simulink model "Demo_PreScanCarSim3D_ExtFMU_cs"  (Simulink 8.6)
settings: Solver=ode5  SolverMode=SingleTasking  StartTime=0.0  StopTime=68  FixedStep=1/1000  RelTol=1e-3
PreLoadFcn:
  | mbxruntime.callbacks.PreLoadFcn(bdroot);
  | check_NUTS_defined;
  | 
  | assignin('base',['model_closed_' bdroot],false);
PostLoadFcn:
  | mbxruntime.callbacks.PostLoadFcn(bdroot);
InitFcn:
  | mbxruntime.callbacks.InitFcn(bdroot);
StartFcn:
  | mbxruntime.callbacks.StartFcn(bdroot);
StopFcn:
  | mbxruntime.callbacks.StopFcn(bdroot);
undefined symbols (not defined in the file): DiscIntNeverNeededParam, mbxruntime, tabledata, warningInitialVelocity, x0, x_ini_VRML, y_ini_VRML, z_ini_VRML
libraries: PreScanSimulinkLibrary x15, simulink_extras x8, simulink x5, PreScanCarSimLibrary x1
(part 2 of 11)

== system Demo_PreScanCarSim3D_ExtFMU_cs/TrafficLightRoadSideNL_1 ==
  DISABLED : Subsystem  VariantControl=off
  ENABLED : Subsystem  VariantControl=on
  VISUCasingLights_TrafficLightRoadSideNL_1 : Outport  Tag=outport/VisuCasingLights  SampleTime=50/1000

== system Demo_PreScanCarSim3D_ExtFMU_cs/TrafficLightRoadSideNL_2 ==
  DISABLED : Subsystem  VariantControl=off
  ENABLED : Subsystem  VariantControl=on
  VISUCasingLights_TrafficLightRoadSideNL_2 : Outport  Tag=outport/VisuCasingLights  SampleTime=50/1000

== system Demo_PreScanCarSim3D_ExtFMU_cs/TrafficLightRoadSideNL_3 ==
  DISABLED : Subsystem  VariantControl=off
  ENABLED : Subsystem  VariantControl=on
  VISUCasingLights_TrafficLightRoadSideNL_3 : Outport  Tag=outport/VisuCasingLights  SampleTime=50/1000

== system Demo_PreScanCarSim3D_ExtFMU_cs/TrafficLightRoadSideNL_5 ==
  DISABLED : Subsystem  VariantControl=off
  ENABLED : Subsystem  VariantControl=on
  VISUCasingLights_TrafficLightRoadSideNL_5 : Outport  Tag=outport/VisuCasingLights  SampleTime=50/1000

== system Demo_PreScanCarSim3D_ExtFMU_cs/TrafficLightRoadSideNL_6 ==
  DISABLED : Subsystem  VariantControl=off
  ENABLED : Subsystem  VariantControl=on
  VISUCasingLights_TrafficLightRoadSideNL_6 : Outport  Tag=outport/VisuCasingLights  SampleTime=50/1000

== system Demo_PreScanCarSim3D_ExtFMU_cs/TrafficLightRoadSideNL_7 ==
  DISABLED : Subsystem  VariantControl=off
  ENABLED : Subsystem  VariantControl=on
  VISUCasingLights_TrafficLightRoadSideNL_7 : Outport  Tag=outport/VisuCasingLights  SampleTime=50/1000

== system Demo_PreScanCarSim3D_ExtFMU_cs/VISUCasingLights_TrafficLightRoadSideNL_1 ==
  VISUCasingLights_TrafficLightRoadSideNL_1 : Inport  Tag=inport/VisuCasingLights  SampleTime=50/1000  BusOutputAsStruct=on
  DISABLED : Subsystem  VariantControl=off
  ENABLED : Subsystem  VariantControl=on

== system Demo_PreScanCarSim3D_ExtFMU_cs/VISUCasingLights_TrafficLightRoadSideNL_2 ==
  VISUCasingLights_TrafficLightRoadSideNL_2 : Inport  Tag=inport/VisuCasingLights  SampleTime=50/1000  BusOutputAsStruct=on
  DISABLED : Subsystem  VariantControl=off
  ENABLED : Subsystem  VariantControl=on

== system Demo_PreScanCarSim3D_ExtFMU_cs/VISUCasingLights_TrafficLightRoadSideNL_3 ==
  VISUCasingLights_TrafficLightRoadSideNL_3 : Inport  Tag=inport/VisuCasingLights  SampleTime=50/1000  BusOutputAsStruct=on
  DISABLED : Subsystem  VariantControl=off
  ENABLED : Subsystem  VariantControl=on

== system Demo_PreScanCarSim3D_ExtFMU_cs/VISUCasingLights_TrafficLightRoadSideNL_5 ==
  VISUCasingLights_TrafficLightRoadSideNL_5 : Inport  Tag=inport/VisuCasingLights  SampleTime=50/1000  BusOutputAsStruct=on
  DISABLED : Subsystem  VariantControl=off
  ENABLED : Subsystem  VariantControl=on

== system Demo_PreScanCarSim3D_ExtFMU_cs/VISUCasingLights_TrafficLightRoadSideNL_6 ==
  VISUCasingLights_TrafficLightRoadSideNL_6 : Inport  Tag=inport/VisuCasingLights  SampleTime=50/1000  BusOutputAsStruct=on
  DISABLED : Subsystem  VariantControl=off
  ENABLED : Subsystem  VariantControl=on

== system Demo_PreScanCarSim3D_ExtFMU_cs/VISUCasingLights_TrafficLightRoadSideNL_7 ==
  VISUCasingLights_TrafficLightRoadSideNL_7 : Inport  Tag=inport/VisuCasingLights  SampleTime=50/1000  BusOutputAsStruct=on
  DISABLED : Subsystem  VariantControl=off
  ENABLED : Subsystem  VariantControl=on

== system Demo_PreScanCarSim3D_ExtFMU_cs/VISUMatrixSignLights_HighwayOverhang_1 ==
  VISUMatrixSignLights_HighwayOverhang_1 : Inport  Tag=inport/VisuMatrixSignLights  SampleTime=50/1000  BusOutputAsStruct=on
  DISABLED : Subsystem  VariantControl=off
  ENABLED : Subsystem  VariantControl=on

== system Demo_PreScanCarSim3D_ExtFMU_cs/VISUMatrixSignLights_HighwayOverhang_2 ==
  VISUMatrixSignLights_HighwayOverhang_2 : Inport  Tag=inport/VisuMatrixSignLights  SampleTime=50/1000  BusOutputAsStruct=on
  DISABLED : Subsystem  VariantControl=off
  ENABLED : Subsystem  VariantControl=on

== system Demo_PreScanCarSim3D_ExtFMU_cs/VISUMatrixSignLights_HighwayOverhang_3 ==
  VISUMatrixSignLights_HighwayOverhang_3 : Inport  Tag=inport/VisuMatrixSignLights  SampleTime=50/1000  BusOutputAsStruct=on
  DISABLED : Subsystem  VariantControl=off
  ENABLED : Subsystem  VariantControl=on

== system Demo_PreScanCarSim3D_ExtFMU_cs/VISUMatrixSignLights_HighwayOverhang_5 ==
  VISUMatrixSignLights_HighwayOverhang_5 : Inport  Tag=inport/VisuMatrixSignLights  SampleTime=50/1000  BusOutputAsStruct=on
  DISABLED : Subsystem  VariantControl=off
  ENABLED : Subsystem  VariantControl=on

== system Demo_PreScanCarSim3D_ExtFMU_cs/VISUMatrixSign_HighwayOverhang_1 ==
  VISUMatrixSign_HighwayOverhang_1 : Inport  Tag=inport/VisuMatrixSign  SampleTime=50/1000  BusOutputAsStruct=on
  DISABLED : Subsystem  VariantControl=off
  ENABLED : Subsystem  VariantControl=on

== system Demo_PreScanCarSim3D_ExtFMU_cs/VISUMatrixSign_HighwayOverhang_2 ==
  VISUMatrixSign_HighwayOverhang_2 : Inport  Tag=inport/VisuMatrixSign  SampleTime=50/1000  BusOutputAsStruct=on
  DISABLED : Subsystem  VariantControl=off
  ENABLED : Subsystem  VariantControl=on

== system Demo_PreScanCarSim3D_ExtFMU_cs/VISUMatrixSign_HighwayOverhang_3 ==
  VISUMatrixSign_HighwayOverhang_3 : Inport  Tag=inport/VisuMatrixSign  SampleTime=50/1000  BusOutputAsStruct=on
  DISABLED : Subsystem  VariantControl=off
  ENABLED : Subsystem  VariantControl=on

== system Demo_PreScanCarSim3D_ExtFMU_cs/VISUMatrixSign_HighwayOverhang_5 ==
  VISUMatrixSign_HighwayOverhang_5 : Inport  Tag=inport/VisuMatrixSign  SampleTime=50/1000  BusOutputAsStruct=on
  DISABLED : Subsystem  VariantControl=off
  ENABLED : Subsystem  VariantControl=on

== system Demo_PreScanCarSim3D_ExtFMU_cs/VISUWheelsCarSim_Audi_A8_1 ==
  VISUWheelsCarSim_Audi_A8_1 : Inport  Tag=inport/VisuWheels  SampleTime=50/1000  BusOutputAsStruct=on
  DISABLED : Subsystem  VariantControl=off
  ENABLED : Subsystem  VariantControl=on

== system Demo_PreScanCarSim3D_ExtFMU_cs/Audi_A8_1/DISABLED ==
  SELF_Audi_A8_1 : Inport  Tag=inport/SelfPort  OutDataTypeStr=Bus: PRESCAN_SELFSENSORDATA  PortDimensions=1  SampleTime=50/1000  BusOutputAsStruct=on
  FromCarSimFMU : Inport  Tag=inport/  Port=2  BusOutputAsStruct=on
  GND1 : Subsystem
  GND2 : Ground
  GND3 : Ground
  TRM1 : Terminator
  TRM2 : Terminator
  STATE_Audi_A8_1_bus : Outport  Tag=outport/StatePort  OutDataTypeStr=Bus: PRESCAN_STATEACTUATORDATA  PortDimensions=1  SampleTime=50/1000
  VISUWheelsCarSim_Audi_A8_1 : Outport  Tag=outport/VisuWheels  Port=2  SampleTime=50/1000
  ToCarSimFMU : Outport  Tag=outport/  Port=3
  wires:
  SELF_Audi_A8_1/1 -> TRM1/1
  FromCarSimFMU/1 -> TRM2/1
  GND1/1(bus) -> STATE_Audi_A8_1_bus/1
  GND2/1 -> VISUWheelsCarSim_Audi_A8_1/1
  GND3/1 -> ToCarSimFMU/1

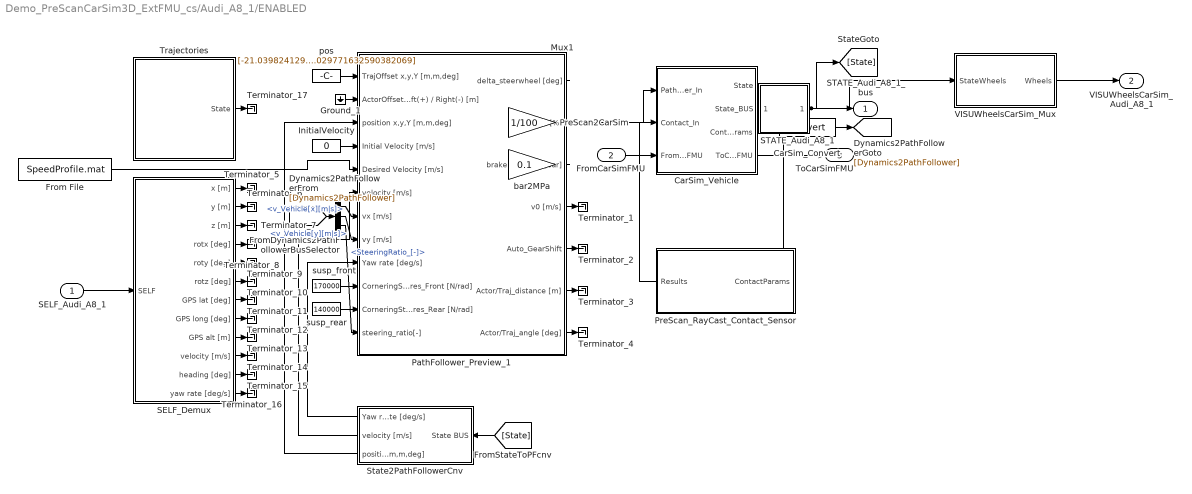
== system Demo_PreScanCarSim3D_ExtFMU_cs/Audi_A8_1/ENABLED ==
  SELF_Audi_A8_1 : Inport  Tag=inport/SelfPort  OutDataTypeStr=Bus: PRESCAN_SELFSENSORDATA  PortDimensions=1  SampleTime=50/1000  BusOutputAsStruct=on
  FromCarSimFMU : Inport  Port=2
  CarSim_Convert : PreScanCarSimLibrary/Convert  Tag=ConvertCarSim  SystemSampleTime=-1
  CarSim_Vehicle : Subsystem  Tag=UserSpecified_Subsys  Description=.\Connection2CarSimFMU.mdl  mask(User specified subsystem){update=off, sourcefilename=.\Connection2CarSimFMU.mdl}
      mask prompts: update "Update (default: not checked)"; sourcefilename "Source file name"
      mask help:
      | A User-specified model may be selected as Controller or Dynamics of the vehicle. PreScan will copy the contents of the User-specified model into the user-specified model block.
      |
      | If update checkbox is checked the current user-specified model block will be deleted and will be REPLACED by (new) user specified model blocks. So, the current user specified model elements will be lost.
      |
      | Warning: If a new user-specified model is selected in the GUI, the user-specified model will be replaced.
      settings: DeleteFcn=PreScanBlockDeleteFcn;
      mask Help: eval('openHelp(227)')
      mask Display: userSpecifiedDynamics_mask_display();
  From File : FromFile  FileName=SpeedProfile.mat  SampleTime=eval(get_param(bdroot,'FixedStep'))
  FromDynamics2PathFollowerBusSelector : BusSelector  OutputSignals=v_Vehicle[x][m|s],v_Vehicle[y][m|s],SteeringRatio_[-]
  Ground_1 : Ground
  InitialVelocity : Constant  Tag=InitialVelocity  Value=0
  Mux1 : Mux  Inputs=3
  PathFollower_Preview_1 : Subsystem  Tag=PathFollower_Preview  mask(PreScan Block: Path Follower with Preview){Migrate=on, FileName='Trajectory_1.mat', mass=1820, Jzz=4095, length_a=1.265, length_l=2.947, Angle_Max_SteeringWheel=500, PreviewTime=0.8, DelayTime=0.1, LowSpeedLimit=20, MaxSteeringRate=1200, CSSampleTime=1/1000, PFIntegrationFrequency=250}
      mask prompts: Migrate "Migrate. During migration this block will be replaced by a newer one."; FileName "Trajectory Name"; mass "Mass vehicle total [kg]"; Jzz "Inertia vehicle around yaw axis [kg m2]"; length_a "Distance between COG and front axle [m]"; length_l "Length of wheelbase [m]"; Angle_Max_SteeringWheel "Maximum steering wheel angle [deg]"; PreviewTime "Preview time [s]"; DelayTime "Delay time [s]"; LowSpeedLimit "Low-speed limit [km/h]"; MaxSteeringRate "Maximum steering wheel angle rate [deg/s]"; CSSampleTime "Compilation Sheet sample time [s]"; PFIntegrationFrequency "Lateral controller frequency [Hz]"
      mask help:
      | The Path Follower Model is selected in the GUI to simulate driver behavior.
      |
      | For more information, please click Help.
      mask init:
      | load(['trajectories/',eval(FileName)])
      | traject=trajectory';
      | 
      | Traj_x=traject(:,2);
      | Traj_y=traject(:,3);
      | Traj_t=traject(2,1);
      | Traj_v=sqrt(traject(:,8).^2+traject(:,9).^2+traject(:,10).^2);
      | 
      | RefreshCounter = (1/CSSampleTime) / (PFIntegrationFrequency); %Compilation sheet frequency/path follower frequency
      | 
      | blockPath = gcb;
      | 
      | clear traject;
      mask Help: eval('openHelp(233)')
  PreScan2CarSim : Gain  Gain=1/100
  PreScan_RayCast_Contact_Sensor : Subsystem  Tag=PreScan_RayCast_Contact_Sensor  LoadFcn=|  mask(PreScan Block: PreScan RayCast Contact Sensor){x0=-21.039824129566149, y0=-15.143190800389089, z0=0, Roll0=0, Pitch0=0, Yaw0=0.029771632590382069, wheelRadius=0.358, hcog=0, b=2.947, TimeStep=-1}
      | load PrescanXYZData;
      | load PrescanRPYData;
      | load PrescanQuatData;
      | load PrescanAxisAngleData;
      | load PrescanPoseData;
      | load PrescanPoseQData;
      | load PrescanPoseAData;
      | load PrescanWheelContactData;
      mask prompts: x0 "Ini x-position VEHICLE wrt GLOBAL axis system [m]"; y0 "Ini y-position VEHICLE wrt GLOBAL axis system [m]"; z0 "Ini z-position VEHICLE wrt GLOBAL axis system [m]"; Roll0 "Ini roll-angle BODY wrt VEHICLE axis system [deg]"; Pitch0 "Ini pitch-angle BODY wrt VEHICLE axis system [deg]"; Yaw0 "Ini yaw-angle VEHICLE wrt GLOBAL axis system [deg]"; wheelRadius "Wheel Radius [m]"; hcog "Dynamics: hCoG [m]"; b "Dynamics: b [m]"; TimeStep "Time Step [s]"
      mask help:
      | This block encapsulates the base Contact sensor.
      |
      | It takes input parameters from the PreScan 3D vehicle dynamics block and outputs contact results.
      mask Help: eval('openHelp(251)')
  SELF_Demux : Subsystem  Tag=demux/SelfPort  mask(PreScan Demux Block:){}
      mask help:
      | The SELF port shows (state) information of the actor itself. The outputs are position in the experiment's axis system and the GPS coordinates, and the object's absolute velocity and compass heading.
      |
      | For more information, please click Help.
      settings: DeleteFcn=PreScanBlockDeleteFcn;
      mask Help: eval('openHelp(462)')
      mask Display:
      | port_label('output',1,'x [m]')
      | port_label('output',2,'y [m]')
      | port_label('output',3,'z [m]','texmode','on')
      | port_label('output',4,'Rotx [deg]','texmode','on')
      | port_label('output',5,'Roty [deg]','texmode','on')
      | port_label('output',6,'Rotz [deg]','texmode','on')
      | port_label('output',7,'GPS lat [deg]','texmode','on')
      | port_label('output',8,'GPS long [deg]','texmode','on')
      | port_label('output',9,'GPS alt [m]','texmode','on')
      | port_label('output',10,'Velocity [m/s]')
      | port_label('output',11,'Heading [deg]')
      | port_label('output',12,'Yaw rate [deg/s]')
  STATE_Audi_A8_1 : Subsystem  Tag=mux/StatePort  Priority=0  LoadFcn=load PrescanStateActuatorData  mask(PreScan Sink Block: State){x0=-21.039824129566149, y0=-15.143190800389089, z0=0, Roll0=0, Pitch0=0, Yaw0=0.029771632590382069, TimeStep=1/1000}
      mask prompts: x0 "Ini x-position VEHICLE wrt GLOBAL axis system [m]"; y0 "Ini y-position VEHICLE wrt GLOBAL axis system [m]"; z0 "Ini z-position VEHICLE wrt GLOBAL axis system [m]"; Roll0 "Ini roll-angle BODY wrt VEHICLE axis system [deg]"; Pitch0 "Ini pitch-angle BODY wrt VEHICLE axis system [deg]"; Yaw0 "Ini yaw-angle VEHICLE wrt GLOBAL axis system [deg]"; TimeStep "Auto-Assigned: Upload Period [s]"
      mask help:
      | The Actor State contains a vector signal of size (9x1), containing the following signals:
      |
      | -  Position                  (x,y,z)                                     [m]
      | -  Velocity                  (vx,vy,vz)                               [m/s]
      | -  Angles                    (Roll, Pitch, Yaw)                   [rad]
      |
      | The Actor state is defined in the global axis system.
      | The state is superponed on the Initial position defined in the GUI.
      |
      | For more information, please click Help.
      settings: DeleteFcn=PreScanBlockDeleteFcn;
      mask Help: eval('openHelp(222)')
      mask Display: image(imread('State.png'))
  State2PathFollowerCnv : Subsystem  Tag=State2PFConnection/cnv
  Terminator_{1..17} (17 alike) : Terminator
  Trajectories : Subsystem  Tag=Trajectories  mask(PreScan Source Block: Trajectories){}
      mask help:
      | The Trajectory block contains the trajectories defined in the PreScan Experiment Editor. The output of the trajectory block is the (vehicle) State.
      |
      | For more information, please click Help.
      settings: DeleteFcn=PreScanBlockDeleteFcn;
      mask Help: eval('openHelp(312)')
      mask Display: image(imread('Trajectory.png'));
  VISUWheelsCarSim_Mux : Subsystem  Tag=MuxWheelsCarSim  mask(PreScan User Interface: VisuWheels){TimeStep=50/1000}
      mask prompts: TimeStep "Auto Assigned: Time Step [s]"
      mask help:
      | The VisuWheels block provides a way to animate the wheels of a vehicle, with steering, rotation (because of velocity) and z-displacement.
      |
      | For more information, please click Help.
      settings: DeleteFcn=PreScanBlockDeleteFcn;
      mask Help: eval('openHelp(223)')
  bar2MPa : Gain  Gain=0.1
  pos : Constant  Tag=pos  Value=[-21.039824129566149 -15.143190800389089 0.029771632590382069]
  susp_front : Constant  Tag=susp_front  Value=170000
  susp_rear : Constant  Tag=susp_rear  Value=140000
  STATE_Audi_A8_1_bus : Outport  Tag=outport/StatePort  OutDataTypeStr=Bus: PRESCAN_STATEACTUATORDATA  PortDimensions=1  SampleTime=50/1000
  VISUWheelsCarSim_Audi_A8_1 : Outport  Tag=outport/VisuWheels  Port=2  SampleTime=50/1000
  ToCarSimFMU : Outport  Port=3
  wires:
  FromCarSimFMU/1 -> CarSim_Vehicle/3(FromCarSimFMU)
  From File/1 -> PathFollower_Preview_1/5(Desired Velocity [m/s])
  CarSim_Vehicle/4(ToCarSimFMU) -> ToCarSimFMU/1
  PreScan2CarSim/1 -> Mux1/2
  bar2MPa/1 -> Mux1/3
  Mux1/1 -> CarSim_Vehicle/1(PathFollower_In)
  PathFollower_Preview_1/1(delta_steerwheel [deg]) -> Mux1/1
  PathFollower_Preview_1/2(throttle [%]) -> PreScan2CarSim/1
  PathFollower_Preview_1/3(brake pressure [bar]) -> bar2MPa/1
  STATE_Audi_A8_1/1(StateBus) -> STATE_Audi_A8_1_bus/1, [State]
  SELF_Audi_A8_1/1 -> SELF_Demux/1(SELF)
  VISUWheelsCarSim_Mux/1(Wheels) -> VISUWheelsCarSim_Audi_A8_1/1
  CarSim_Vehicle/3(ContactParams) -> PreScan_RayCast_Contact_Sensor/1(ContactParams)
  PreScan_RayCast_Contact_Sensor/1(Results) -> CarSim_Vehicle/2(Contact_In)
  CarSim_Vehicle/2(State_BUS) -> VISUWheelsCarSim_Mux/1(StateWheels), CarSim_Convert/1
  pos/1 -> PathFollower_Preview_1/1(TrajOffset x,y,Y [m,m,deg])
  susp_front/1 -> PathFollower_Preview_1/10(CorneringStiffness_Tyres_Front [N/rad])
  susp_rear/1 -> PathFollower_Preview_1/11(CorneringStiffness_Tyres_Rear [N/rad])
  InitialVelocity/1 -> PathFollower_Preview_1/4(Initial Velocity [m/s])
  [State] -> State2PathFollowerCnv/1(State BUS)
  State2PathFollowerCnv/1(Yaw rate [deg/s]) -> PathFollower_Preview_1/9(Yaw rate [deg/s])
  State2PathFollowerCnv/2(velocity [m/s]) -> PathFollower_Preview_1/6(velocity [m/s])
  State2PathFollowerCnv/3(position x,y,Y [m,m,deg]) -> PathFollower_Preview_1/3(position x,y,Y [m,m,deg])
  CarSim_Convert/1 -> [Dynamics2PathFollower]
  FromDynamics2PathFollowerBusSelector/1 -> PathFollower_Preview_1/7(vx [m/s])  "<v_Vehicle[x][m|s]>"
  FromDynamics2PathFollowerBusSelector/2 -> PathFollower_Preview_1/8(vy [m/s])  "<v_Vehicle[y][m|s]>"
  FromDynamics2PathFollowerBusSelector/3 -> PathFollower_Preview_1/12(steering_ratio[-])  "<SteeringRatio_[-]>"
  [Dynamics2PathFollower] -> FromDynamics2PathFollowerBusSelector/1
  CarSim_Vehicle/1(State) -> STATE_Audi_A8_1/1(State)
  Ground_1/1 -> PathFollower_Preview_1/2(ActorOffset_Left(+) / Right(-) [m])
  PathFollower_Preview_1/4(v0 [m/s]) -> Terminator_1/1
  PathFollower_Preview_1/5(Auto_GearShift) -> Terminator_2/1
  PathFollower_Preview_1/6(Actor/Traj_distance [m]) -> Terminator_3/1
  PathFollower_Preview_1/7(Actor/Traj_angle [deg]) -> Terminator_4/1
  SELF_Demux/1(x [m]) -> Terminator_5/1
  SELF_Demux/2(y [m]) -> Terminator_6/1
  SELF_Demux/3(z [m]) -> Terminator_7/1
  SELF_Demux/4(rotx [deg]) -> Terminator_8/1
  SELF_Demux/5(roty [deg]) -> Terminator_9/1
  SELF_Demux/6(rotz [deg]) -> Terminator_10/1
  SELF_Demux/7(GPS lat [deg]) -> Terminator_11/1
  SELF_Demux/8(GPS long [deg]) -> Terminator_12/1
  SELF_Demux/9(GPS alt [m]) -> Terminator_13/1
  SELF_Demux/10(velocity [m/s]) -> Terminator_14/1
  SELF_Demux/11(heading [deg]) -> Terminator_15/1
  SELF_Demux/12(yaw rate [deg/s]) -> Terminator_16/1
  Trajectories/1(State) -> Terminator_17/1

== system Demo_PreScanCarSim3D_ExtFMU_cs/Box_1/DISABLED ==
  SELF_Box_1 : Inport  Tag=inport/SelfPort  OutDataTypeStr=Bus: PRESCAN_SELFSENSORDATA  PortDimensions=1  SampleTime=50/1000  BusOutputAsStruct=on
  GND1 : Subsystem
  TRM1 : Terminator
  STATE_Box_1_bus : Outport  Tag=outport/StatePort  OutDataTypeStr=Bus: PRESCAN_STATEACTUATORDATA  PortDimensions=1  SampleTime=50/1000
  wires:
  SELF_Box_1/1 -> TRM1/1
  GND1/1(bus) -> STATE_Box_1_bus/1

== system Demo_PreScanCarSim3D_ExtFMU_cs/Box_1/ENABLED ==
  SELF_Box_1 : Inport  Tag=inport/SelfPort  OutDataTypeStr=Bus: PRESCAN_SELFSENSORDATA  PortDimensions=1  SampleTime=50/1000  BusOutputAsStruct=on
  Dynamics_Empty : Subsystem  Tag=Dynamics_Empty
      mask Help: eval('openHelp(202)')
      mask Display: port_label('output', 1, 'State');text(0,0,' Empty\n')
  SELF_Demux : Subsystem  Tag=demux/SelfPort  mask(PreScan Demux Block:){}
      mask help:
      | The SELF port shows (state) information of the actor itself. The outputs are position in the experiment's axis system and the GPS coordinates, and the object's absolute velocity and compass heading.
      |
      | For more information, please click Help.
      settings: DeleteFcn=PreScanBlockDeleteFcn;
      mask Help: eval('openHelp(462)')
      mask Display:
      | port_label('output',1,'x [m]')
      | port_label('output',2,'y [m]')
      | port_label('output',3,'z [m]','texmode','on')
      | port_label('output',4,'Rotx [deg]','texmode','on')
      | port_label('output',5,'Roty [deg]','texmode','on')
      | port_label('output',6,'Rotz [deg]','texmode','on')
      | port_label('output',7,'GPS lat [deg]','texmode','on')
      | port_label('output',8,'GPS long [deg]','texmode','on')
      | port_label('output',9,'GPS alt [m]','texmode','on')
      | port_label('output',10,'Velocity [m/s]')
      | port_label('output',11,'Heading [deg]')
      | port_label('output',12,'Yaw rate [deg/s]')
  STATE_Box_1 : Subsystem  Tag=mux/StatePort  Priority=0  LoadFcn=load PrescanStateActuatorData  mask(PreScan Sink Block: State){x0=340, y0=0, z0=2.45, Roll0=0, Pitch0=0, Yaw0=0, TimeStep=1/1000}
      mask prompts: x0 "Ini x-position VEHICLE wrt GLOBAL axis system [m]"; y0 "Ini y-position VEHICLE wrt GLOBAL axis system [m]"; z0 "Ini z-position VEHICLE wrt GLOBAL axis system [m]"; Roll0 "Ini roll-angle BODY wrt VEHICLE axis system [deg]"; Pitch0 "Ini pitch-angle BODY wrt VEHICLE axis system [deg]"; Yaw0 "Ini yaw-angle VEHICLE wrt GLOBAL axis system [deg]"; TimeStep "Auto-Assigned: Upload Period [s]"
      mask help:
      | The Actor State contains a vector signal of size (9x1), containing the following signals:
      |
      | -  Position                  (x,y,z)                                     [m]
      | -  Velocity                  (vx,vy,vz)                               [m/s]
      | -  Angles                    (Roll, Pitch, Yaw)                   [rad]
      |
      | The Actor state is defined in the global axis system.
      | The state is superponed on the Initial position defined in the GUI.
      |
      | For more information, please click Help.
      settings: DeleteFcn=PreScanBlockDeleteFcn;
      mask Help: eval('openHelp(222)')
      mask Display: image(imread('State.png'))
  Terminator_{1..12} (12 alike) : Terminator
  STATE_Box_1_bus : Outport  Tag=outport/StatePort  OutDataTypeStr=Bus: PRESCAN_STATEACTUATORDATA  PortDimensions=1  SampleTime=50/1000
  wires:
  STATE_Box_1/1(StateBus) -> STATE_Box_1_bus/1
  SELF_Box_1/1 -> SELF_Demux/1(SELF)
  Dynamics_Empty/1(State) -> STATE_Box_1/1(State)
  SELF_Demux/1(x [m]) -> Terminator_1/1
  SELF_Demux/2(y [m]) -> Terminator_2/1
  SELF_Demux/3(z [m]) -> Terminator_3/1
  SELF_Demux/4(rotx [deg]) -> Terminator_4/1
  SELF_Demux/5(roty [deg]) -> Terminator_5/1
  SELF_Demux/6(rotz [deg]) -> Terminator_6/1
  SELF_Demux/7(GPS lat [deg]) -> Terminator_7/1
  SELF_Demux/8(GPS long [deg]) -> Terminator_8/1
  SELF_Demux/9(GPS alt [m]) -> Terminator_9/1
  SELF_Demux/10(velocity [m/s]) -> Terminator_10/1
  SELF_Demux/11(heading [deg]) -> Terminator_11/1
  SELF_Demux/12(yaw rate [deg/s]) -> Terminator_12/1

== system Demo_PreScanCarSim3D_ExtFMU_cs/Box_2/DISABLED ==
  SELF_Box_2 : Inport  Tag=inport/SelfPort  OutDataTypeStr=Bus: PRESCAN_SELFSENSORDATA  PortDimensions=1  SampleTime=50/1000  BusOutputAsStruct=on
  GND1 : Subsystem
  TRM1 : Terminator
  STATE_Box_2_bus : Outport  Tag=outport/StatePort  OutDataTypeStr=Bus: PRESCAN_STATEACTUATORDATA  PortDimensions=1  SampleTime=50/1000
  wires:
  SELF_Box_2/1 -> TRM1/1
  GND1/1(bus) -> STATE_Box_2_bus/1

== system Demo_PreScanCarSim3D_ExtFMU_cs/Box_2/ENABLED ==
  SELF_Box_2 : Inport  Tag=inport/SelfPort  OutDataTypeStr=Bus: PRESCAN_SELFSENSORDATA  PortDimensions=1  SampleTime=50/1000  BusOutputAsStruct=on
  Dynamics_Empty : Subsystem  Tag=Dynamics_Empty
      mask Help: eval('openHelp(202)')
      mask Display: port_label('output', 1, 'State');text(0,0,' Empty\n')
  SELF_Demux : Subsystem  Tag=demux/SelfPort  mask(PreScan Demux Block:){}
      mask help:
      | The SELF port shows (state) information of the actor itself. The outputs are position in the experiment's axis system and the GPS coordinates, and the object's absolute velocity and compass heading.
      |
      | For more information, please click Help.
      settings: DeleteFcn=PreScanBlockDeleteFcn;
      mask Help: eval('openHelp(462)')
      mask Display:
      | port_label('output',1,'x [m]')
      | port_label('output',2,'y [m]')
      | port_label('output',3,'z [m]','texmode','on')
      | port_label('output',4,'Rotx [deg]','texmode','on')
      | port_label('output',5,'Roty [deg]','texmode','on')
      | port_label('output',6,'Rotz [deg]','texmode','on')
      | port_label('output',7,'GPS lat [deg]','texmode','on')
      | port_label('output',8,'GPS long [deg]','texmode','on')
      | port_label('output',9,'GPS alt [m]','texmode','on')
      | port_label('output',10,'Velocity [m/s]')
      | port_label('output',11,'Heading [deg]')
      | port_label('output',12,'Yaw rate [deg/s]')
  STATE_Box_2 : Subsystem  Tag=mux/StatePort  Priority=0  LoadFcn=load PrescanStateActuatorData  mask(PreScan Sink Block: State){x0=345, y0=0, z0=2.45, Roll0=0, Pitch0=0, Yaw0=0, TimeStep=1/1000}
      mask prompts: x0 "Ini x-position VEHICLE wrt GLOBAL axis system [m]"; y0 "Ini y-position VEHICLE wrt GLOBAL axis system [m]"; z0 "Ini z-position VEHICLE wrt GLOBAL axis system [m]"; Roll0 "Ini roll-angle BODY wrt VEHICLE axis system [deg]"; Pitch0 "Ini pitch-angle BODY wrt VEHICLE axis system [deg]"; Yaw0 "Ini yaw-angle VEHICLE wrt GLOBAL axis system [deg]"; TimeStep "Auto-Assigned: Upload Period [s]"
      mask help:
      | The Actor State contains a vector signal of size (9x1), containing the following signals:
      |
      | -  Position                  (x,y,z)                                     [m]
      | -  Velocity                  (vx,vy,vz)                               [m/s]
      | -  Angles                    (Roll, Pitch, Yaw)                   [rad]
      |
      | The Actor state is defined in the global axis system.
      | The state is superponed on the Initial position defined in the GUI.
      |
      | For more information, please click Help.
      settings: DeleteFcn=PreScanBlockDeleteFcn;
      mask Help: eval('openHelp(222)')
      mask Display: image(imread('State.png'))
  Terminator_{1..12} (12 alike) : Terminator
  STATE_Box_2_bus : Outport  Tag=outport/StatePort  OutDataTypeStr=Bus: PRESCAN_STATEACTUATORDATA  PortDimensions=1  SampleTime=50/1000
  wires:
  STATE_Box_2/1(StateBus) -> STATE_Box_2_bus/1
  SELF_Box_2/1 -> SELF_Demux/1(SELF)
  Dynamics_Empty/1(State) -> STATE_Box_2/1(State)
  SELF_Demux/1(x [m]) -> Terminator_1/1
  SELF_Demux/2(y [m]) -> Terminator_2/1
  SELF_Demux/3(z [m]) -> Terminator_3/1
  SELF_Demux/4(rotx [deg]) -> Terminator_4/1
  SELF_Demux/5(roty [deg]) -> Terminator_5/1
  SELF_Demux/6(rotz [deg]) -> Terminator_6/1
  SELF_Demux/7(GPS lat [deg]) -> Terminator_7/1
  SELF_Demux/8(GPS long [deg]) -> Terminator_8/1
  SELF_Demux/9(GPS alt [m]) -> Terminator_9/1
  SELF_Demux/10(velocity [m/s]) -> Terminator_10/1
  SELF_Demux/11(heading [deg]) -> Terminator_11/1
  SELF_Demux/12(yaw rate [deg/s]) -> Terminator_12/1

== system Demo_PreScanCarSim3D_ExtFMU_cs/Box_3/DISABLED ==
  SELF_Box_3 : Inport  Tag=inport/SelfPort  OutDataTypeStr=Bus: PRESCAN_SELFSENSORDATA  PortDimensions=1  SampleTime=50/1000  BusOutputAsStruct=on
  GND1 : Subsystem
  TRM1 : Terminator
  STATE_Box_3_bus : Outport  Tag=outport/StatePort  OutDataTypeStr=Bus: PRESCAN_STATEACTUATORDATA  PortDimensions=1  SampleTime=50/1000
  wires:
  SELF_Box_3/1 -> TRM1/1
  GND1/1(bus) -> STATE_Box_3_bus/1

== system Demo_PreScanCarSim3D_ExtFMU_cs/Box_3/ENABLED ==
  SELF_Box_3 : Inport  Tag=inport/SelfPort  OutDataTypeStr=Bus: PRESCAN_SELFSENSORDATA  PortDimensions=1  SampleTime=50/1000  BusOutputAsStruct=on
  Dynamics_Empty : Subsystem  Tag=Dynamics_Empty
      mask Help: eval('openHelp(202)')
      mask Display: port_label('output', 1, 'State');text(0,0,' Empty\n')
  SELF_Demux : Subsystem  Tag=demux/SelfPort  mask(PreScan Demux Block:){}
      mask help:
      | The SELF port shows (state) information of the actor itself. The outputs are position in the experiment's axis system and the GPS coordinates, and the object's absolute velocity and compass heading.
      |
      | For more information, please click Help.
      settings: DeleteFcn=PreScanBlockDeleteFcn;
      mask Help: eval('openHelp(462)')
      mask Display:
      | port_label('output',1,'x [m]')
      | port_label('output',2,'y [m]')
      | port_label('output',3,'z [m]','texmode','on')
      | port_label('output',4,'Rotx [deg]','texmode','on')
      | port_label('output',5,'Roty [deg]','texmode','on')
      | port_label('output',6,'Rotz [deg]','texmode','on')
      | port_label('output',7,'GPS lat [deg]','texmode','on')
      | port_label('output',8,'GPS long [deg]','texmode','on')
      | port_label('output',9,'GPS alt [m]','texmode','on')
      | port_label('output',10,'Velocity [m/s]')
      | port_label('output',11,'Heading [deg]')
      | port_label('output',12,'Yaw rate [deg/s]')
  STATE_Box_3 : Subsystem  Tag=mux/StatePort  Priority=0  LoadFcn=load PrescanStateActuatorData  mask(PreScan Sink Block: State){x0=350, y0=0, z0=2.45, Roll0=0, Pitch0=0, Yaw0=0, TimeStep=1/1000}
      mask prompts: x0 "Ini x-position VEHICLE wrt GLOBAL axis system [m]"; y0 "Ini y-position VEHICLE wrt GLOBAL axis system [m]"; z0 "Ini z-position VEHICLE wrt GLOBAL axis system [m]"; Roll0 "Ini roll-angle BODY wrt VEHICLE axis system [deg]"; Pitch0 "Ini pitch-angle BODY wrt VEHICLE axis system [deg]"; Yaw0 "Ini yaw-angle VEHICLE wrt GLOBAL axis system [deg]"; TimeStep "Auto-Assigned: Upload Period [s]"
      mask help:
      | The Actor State contains a vector signal of size (9x1), containing the following signals:
      |
      | -  Position                  (x,y,z)                                     [m]
      | -  Velocity                  (vx,vy,vz)                               [m/s]
      | -  Angles                    (Roll, Pitch, Yaw)                   [rad]
      |
      | The Actor state is defined in the global axis system.
      | The state is superponed on the Initial position defined in the GUI.
      |
      | For more information, please click Help.
      settings: DeleteFcn=PreScanBlockDeleteFcn;
      mask Help: eval('openHelp(222)')
      mask Display: image(imread('State.png'))
  Terminator_{1..12} (12 alike) : Terminator
  STATE_Box_3_bus : Outport  Tag=outport/StatePort  OutDataTypeStr=Bus: PRESCAN_STATEACTUATORDATA  PortDimensions=1  SampleTime=50/1000
  wires:
  STATE_Box_3/1(StateBus) -> STATE_Box_3_bus/1
  SELF_Box_3/1 -> SELF_Demux/1(SELF)
  Dynamics_Empty/1(State) -> STATE_Box_3/1(State)
  SELF_Demux/1(x [m]) -> Terminator_1/1
  SELF_Demux/2(y [m]) -> Terminator_2/1
  SELF_Demux/3(z [m]) -> Terminator_3/1
  SELF_Demux/4(rotx [deg]) -> Terminator_4/1
  SELF_Demux/5(roty [deg]) -> Terminator_5/1
  SELF_Demux/6(rotz [deg]) -> Terminator_6/1
  SELF_Demux/7(GPS lat [deg]) -> Terminator_7/1
  SELF_Demux/8(GPS long [deg]) -> Terminator_8/1
  SELF_Demux/9(GPS alt [m]) -> Terminator_9/1
  SELF_Demux/10(velocity [m/s]) -> Terminator_10/1
  SELF_Demux/11(heading [deg]) -> Terminator_11/1
  SELF_Demux/12(yaw rate [deg/s]) -> Terminator_12/1

== system Demo_PreScanCarSim3D_ExtFMU_cs/Box_4/DISABLED ==
  SELF_Box_4 : Inport  Tag=inport/SelfPort  OutDataTypeStr=Bus: PRESCAN_SELFSENSORDATA  PortDimensions=1  SampleTime=50/1000  BusOutputAsStruct=on
  GND1 : Subsystem
  TRM1 : Terminator
  STATE_Box_4_bus : Outport  Tag=outport/StatePort  OutDataTypeStr=Bus: PRESCAN_STATEACTUATORDATA  PortDimensions=1  SampleTime=50/1000
  wires:
  SELF_Box_4/1 -> TRM1/1
  GND1/1(bus) -> STATE_Box_4_bus/1

== system Demo_PreScanCarSim3D_ExtFMU_cs/Box_4/ENABLED ==
  SELF_Box_4 : Inport  Tag=inport/SelfPort  OutDataTypeStr=Bus: PRESCAN_SELFSENSORDATA  PortDimensions=1  SampleTime=50/1000  BusOutputAsStruct=on
  Dynamics_Empty : Subsystem  Tag=Dynamics_Empty
      mask Help: eval('openHelp(202)')
      mask Display: port_label('output', 1, 'State');text(0,0,' Empty\n')
  SELF_Demux : Subsystem  Tag=demux/SelfPort  mask(PreScan Demux Block:){}
      mask help:
      | The SELF port shows (state) information of the actor itself. The outputs are position in the experiment's axis system and the GPS coordinates, and the object's absolute velocity and compass heading.
      |
      | For more information, please click Help.
      settings: DeleteFcn=PreScanBlockDeleteFcn;
      mask Help: eval('openHelp(462)')
      mask Display:
      | port_label('output',1,'x [m]')
      | port_label('output',2,'y [m]')
      | port_label('output',3,'z [m]','texmode','on')
      | port_label('output',4,'Rotx [deg]','texmode','on')
      | port_label('output',5,'Roty [deg]','texmode','on')
      | port_label('output',6,'Rotz [deg]','texmode','on')
      | port_label('output',7,'GPS lat [deg]','texmode','on')
      | port_label('output',8,'GPS long [deg]','texmode','on')
      | port_label('output',9,'GPS alt [m]','texmode','on')
      | port_label('output',10,'Velocity [m/s]')
      | port_label('output',11,'Heading [deg]')
      | port_label('output',12,'Yaw rate [deg/s]')
  STATE_Box_4 : Subsystem  Tag=mux/StatePort  Priority=0  LoadFcn=load PrescanStateActuatorData  mask(PreScan Sink Block: State){x0=345, y0=0, z0=4.55, Roll0=0, Pitch0=0, Yaw0=0, TimeStep=1/1000}
      mask prompts: x0 "Ini x-position VEHICLE wrt GLOBAL axis system [m]"; y0 "Ini y-position VEHICLE wrt GLOBAL axis system [m]"; z0 "Ini z-position VEHICLE wrt GLOBAL axis system [m]"; Roll0 "Ini roll-angle BODY wrt VEHICLE axis system [deg]"; Pitch0 "Ini pitch-angle BODY wrt VEHICLE axis system [deg]"; Yaw0 "Ini yaw-angle VEHICLE wrt GLOBAL axis system [deg]"; TimeStep "Auto-Assigned: Upload Period [s]"
      mask help:
      | The Actor State contains a vector signal of size (9x1), containing the following signals:
      |
      | -  Position                  (x,y,z)                                     [m]
      | -  Velocity                  (vx,vy,vz)                               [m/s]
      | -  Angles                    (Roll, Pitch, Yaw)                   [rad]
      |
      | The Actor state is defined in the global axis system.
      | The state is superponed on the Initial position defined in the GUI.
      |
      | For more information, please click Help.
      settings: DeleteFcn=PreScanBlockDeleteFcn;
      mask Help: eval('openHelp(222)')
      mask Display: image(imread('State.png'))
  Terminator_{1..12} (12 alike) : Terminator
  STATE_Box_4_bus : Outport  Tag=outport/StatePort  OutDataTypeStr=Bus: PRESCAN_STATEACTUATORDATA  PortDimensions=1  SampleTime=50/1000
  wires:
  STATE_Box_4/1(StateBus) -> STATE_Box_4_bus/1
  SELF_Box_4/1 -> SELF_Demux/1(SELF)
  Dynamics_Empty/1(State) -> STATE_Box_4/1(State)
  SELF_Demux/1(x [m]) -> Terminator_1/1
  SELF_Demux/2(y [m]) -> Terminator_2/1
  SELF_Demux/3(z [m]) -> Terminator_3/1
  SELF_Demux/4(rotx [deg]) -> Terminator_4/1
  SELF_Demux/5(roty [deg]) -> Terminator_5/1
  SELF_Demux/6(rotz [deg]) -> Terminator_6/1
  SELF_Demux/7(GPS lat [deg]) -> Terminator_7/1
  SELF_Demux/8(GPS long [deg]) -> Terminator_8/1
  SELF_Demux/9(GPS alt [m]) -> Terminator_9/1
  SELF_Demux/10(velocity [m/s]) -> Terminator_10/1
  SELF_Demux/11(heading [deg]) -> Terminator_11/1
  SELF_Demux/12(yaw rate [deg/s]) -> Terminator_12/1

== system Demo_PreScanCarSim3D_ExtFMU_cs/HighwayOverhang_1/DISABLED ==
  GND1 : Ground
  GND2 : Ground
  VISUMatrixSign_HighwayOverhang_1 : Outport  Tag=outport/VisuMatrixSign  SampleTime=50/1000
  VISUMatrixSignLights_HighwayOverhang_1 : Outport  Tag=outport/VisuMatrixSignLights  Port=2  SampleTime=50/1000
  wires:
  GND1/1 -> VISUMatrixSign_HighwayOverhang_1/1
  GND2/1 -> VISUMatrixSignLights_HighwayOverhang_1/1

== system Demo_PreScanCarSim3D_ExtFMU_cs/HighwayOverhang_1/ENABLED ==
  note: Resources
      |
      | 3: InformationSign\MatrixSign_Empty.png: MatrixSign Empty
      | 4: InformationSign\MatrixSign_End.png: MatrixSign End
      | 5: InformationSign\MatrixSign_GreenArrow.png: MatrixSign GreenArrow
      | 6: InformationSign\MatrixSign_RedCross.png: MatrixSign RedCross
      | 7: InformationSign\MatrixSign_Speed_50.png: MatrixSign Speed 50
      | 8: InformationSign\MatrixSign_Speed_70.png: MatrixSign Speed 70
      | 9: InformationSign\MatrixSign_Speed_90.png: MatrixSign Speed 90
      | 10: InformationSign\MatrixSign_Speed_120.png: MatrixSign Speed 120
      | 11: InformationSign\MatrixSign_Speed_130.png: MatrixSign Speed 130
      | 12: InformationSign\information.png: information
      | 13: InformationSign\TASS-international-logo.bmp: TASS-international-logo
  Ground_{1..8} (8 alike) : Ground
  VISUMatrixSignLights_Mux : Subsystem  Tag=mux/VisuMatrixSignLights  mask(PreScan User Interface: VisuMatrixSignLights){}
      mask help:
      | The VisuMatrixSignLights block provides a way to switch the lights on the matrix sign board on or off
      |
      | For more information, please click Help.
      mask Help: eval('openHelp(732)')
  VISUMatrixSign_Mux : Subsystem  Tag=mux/MatrixSign_v2  mask(PreScan User Interface: VisuMatrixSign){}
      mask help:
      | The VisuMatrixSign block provides a way to adapt the texture of the plates connected to an overhang, based on Resource IDs of the texture files.
      |
      | For more information, please click Help.
      settings: DeleteFcn=PreScanBlockDeleteFcn;
      mask Help: eval('openHelp(733)')
  VISUMatrixSign_HighwayOverhang_1 : Outport  Tag=outport/VisuMatrixSign  SampleTime=50/1000
  VISUMatrixSignLights_HighwayOverhang_1 : Outport  Tag=outport/VisuMatrixSignLights  Port=2  SampleTime=50/1000
  wires:
  VISUMatrixSign_Mux/1(MatrixSigns) -> VISUMatrixSign_HighwayOverhang_1/1
  VISUMatrixSignLights_Mux/1(VISUMatrixSignLights_HighwayOverhang_1) -> VISUMatrixSignLights_HighwayOverhang_1/1
  Ground_1/1 -> VISUMatrixSignLights_Mux/1(MatrixSign_1)
  Ground_2/1 -> VISUMatrixSignLights_Mux/2(MatrixSign_2)
  Ground_3/1 -> VISUMatrixSignLights_Mux/3(MatrixSign_3)
  Ground_4/1 -> VISUMatrixSignLights_Mux/4(MatrixSign_4)
  Ground_5/1 -> VISUMatrixSign_Mux/1(MatrixSign_1)
  Ground_6/1 -> VISUMatrixSign_Mux/2(MatrixSign_2)
  Ground_7/1 -> VISUMatrixSign_Mux/3(MatrixSign_3)
  Ground_8/1 -> VISUMatrixSign_Mux/4(MatrixSign_4)

== system Demo_PreScanCarSim3D_ExtFMU_cs/HighwayOverhang_2/DISABLED ==
  GND1 : Ground
  GND2 : Ground
  VISUMatrixSign_HighwayOverhang_2 : Outport  Tag=outport/VisuMatrixSign  SampleTime=50/1000
  VISUMatrixSignLights_HighwayOverhang_2 : Outport  Tag=outport/VisuMatrixSignLights  Port=2  SampleTime=50/1000
  wires:
  GND1/1 -> VISUMatrixSign_HighwayOverhang_2/1
  GND2/1 -> VISUMatrixSignLights_HighwayOverhang_2/1

== system Demo_PreScanCarSim3D_ExtFMU_cs/HighwayOverhang_2/ENABLED ==
  note: Resources
      |
      | 3: InformationSign\MatrixSign_Empty.png: MatrixSign Empty
      | 4: InformationSign\MatrixSign_End.png: MatrixSign End
      | 5: InformationSign\MatrixSign_GreenArrow.png: MatrixSign GreenArrow
      | 6: InformationSign\MatrixSign_RedCross.png: MatrixSign RedCross
      | 7: InformationSign\MatrixSign_Speed_50.png: MatrixSign Speed 50
      | 8: InformationSign\MatrixSign_Speed_70.png: MatrixSign Speed 70
      | 9: InformationSign\MatrixSign_Speed_90.png: MatrixSign Speed 90
      | 10: InformationSign\MatrixSign_Speed_120.png: MatrixSign Speed 120
      | 11: InformationSign\MatrixSign_Speed_130.png: MatrixSign Speed 130
      | 12: InformationSign\information.png: information
      | 13: InformationSign\TASS-international-logo.bmp: TASS-international-logo
  Ground_{1..6} (6 alike) : Ground
  VISUMatrixSignLights_Mux : Subsystem  Tag=mux/VisuMatrixSignLights  mask(PreScan User Interface: VisuMatrixSignLights){}
      mask help:
      | The VisuMatrixSignLights block provides a way to switch the lights on the matrix sign board on or off
      |
      | For more information, please click Help.
      mask Help: eval('openHelp(732)')
  VISUMatrixSign_Mux : Subsystem  Tag=mux/MatrixSign_v2  mask(PreScan User Interface: VisuMatrixSign){}
      mask help:
      | The VisuMatrixSign block provides a way to adapt the texture of the plates connected to an overhang, based on Resource IDs of the texture files.
      |
      | For more information, please click Help.
      settings: DeleteFcn=PreScanBlockDeleteFcn;
      mask Help: eval('openHelp(733)')
  VISUMatrixSign_HighwayOverhang_2 : Outport  Tag=outport/VisuMatrixSign  SampleTime=50/1000
  VISUMatrixSignLights_HighwayOverhang_2 : Outport  Tag=outport/VisuMatrixSignLights  Port=2  SampleTime=50/1000
  wires:
  VISUMatrixSign_Mux/1(MatrixSigns) -> VISUMatrixSign_HighwayOverhang_2/1
  VISUMatrixSignLights_Mux/1(VISUMatrixSignLights_HighwayOverhang_2) -> VISUMatrixSignLights_HighwayOverhang_2/1
  Ground_1/1 -> VISUMatrixSignLights_Mux/1(MatrixSign_5)
  Ground_2/1 -> VISUMatrixSignLights_Mux/2(MatrixSign_6)
  Ground_3/1 -> VISUMatrixSignLights_Mux/3(MatrixSign_7)
  Ground_4/1 -> VISUMatrixSign_Mux/1(MatrixSign_5)
  Ground_5/1 -> VISUMatrixSign_Mux/2(MatrixSign_6)
  Ground_6/1 -> VISUMatrixSign_Mux/3(MatrixSign_7)

== system Demo_PreScanCarSim3D_ExtFMU_cs/HighwayOverhang_3/DISABLED ==
  GND1 : Ground
  GND2 : Ground
  VISUMatrixSign_HighwayOverhang_3 : Outport  Tag=outport/VisuMatrixSign  SampleTime=50/1000
  VISUMatrixSignLights_HighwayOverhang_3 : Outport  Tag=outport/VisuMatrixSignLights  Port=2  SampleTime=50/1000
  wires:
  GND1/1 -> VISUMatrixSign_HighwayOverhang_3/1
  GND2/1 -> VISUMatrixSignLights_HighwayOverhang_3/1

== system Demo_PreScanCarSim3D_ExtFMU_cs/HighwayOverhang_3/ENABLED ==
  note: Resources
      |
      | 3: InformationSign\MatrixSign_Empty.png: MatrixSign Empty
      | 4: InformationSign\MatrixSign_End.png: MatrixSign End
      | 5: InformationSign\MatrixSign_GreenArrow.png: MatrixSign GreenArrow
      | 6: InformationSign\MatrixSign_RedCross.png: MatrixSign RedCross
      | 7: InformationSign\MatrixSign_Speed_50.png: MatrixSign Speed 50
      | 8: InformationSign\MatrixSign_Speed_70.png: MatrixSign Speed 70
      | 9: InformationSign\MatrixSign_Speed_90.png: MatrixSign Speed 90
      | 10: InformationSign\MatrixSign_Speed_120.png: MatrixSign Speed 120
      | 11: InformationSign\MatrixSign_Speed_130.png: MatrixSign Speed 130
      | 12: InformationSign\information.png: information
      | 13: InformationSign\TASS-international-logo.bmp: TASS-international-logo
  Ground_{1..6} (6 alike) : Ground
  VISUMatrixSignLights_Mux : Subsystem  Tag=mux/VisuMatrixSignLights  mask(PreScan User Interface: VisuMatrixSignLights){}
      mask help:
      | The VisuMatrixSignLights block provides a way to switch the lights on the matrix sign board on or off
      |
      | For more information, please click Help.
      mask Help: eval('openHelp(732)')
  VISUMatrixSign_Mux : Subsystem  Tag=mux/MatrixSign_v2  mask(PreScan User Interface: VisuMatrixSign){}
      mask help:
      | The VisuMatrixSign block provides a way to adapt the texture of the plates connected to an overhang, based on Resource IDs of the texture files.
      |
      | For more information, please click Help.
      settings: DeleteFcn=PreScanBlockDeleteFcn;
      mask Help: eval('openHelp(733)')
  VISUMatrixSign_HighwayOverhang_3 : Outport  Tag=outport/VisuMatrixSign  SampleTime=50/1000
  VISUMatrixSignLights_HighwayOverhang_3 : Outport  Tag=outport/VisuMatrixSignLights  Port=2  SampleTime=50/1000
  wires:
  VISUMatrixSign_Mux/1(MatrixSigns) -> VISUMatrixSign_HighwayOverhang_3/1
  VISUMatrixSignLights_Mux/1(VISUMatrixSignLights_HighwayOverhang_3) -> VISUMatrixSignLights_HighwayOverhang_3/1
  Ground_1/1 -> VISUMatrixSignLights_Mux/1(MatrixSign_10)
  Ground_2/1 -> VISUMatrixSignLights_Mux/2(MatrixSign_11)
  Ground_3/1 -> VISUMatrixSignLights_Mux/3(MatrixSign_12)
  Ground_4/1 -> VISUMatrixSign_Mux/1(MatrixSign_10)
  Ground_5/1 -> VISUMatrixSign_Mux/2(MatrixSign_11)
  Ground_6/1 -> VISUMatrixSign_Mux/3(MatrixSign_12)

== system Demo_PreScanCarSim3D_ExtFMU_cs/HighwayOverhang_5/DISABLED ==
  GND1 : Ground
  GND2 : Ground
  VISUMatrixSign_HighwayOverhang_5 : Outport  Tag=outport/VisuMatrixSign  SampleTime=50/1000
  VISUMatrixSignLights_HighwayOverhang_5 : Outport  Tag=outport/VisuMatrixSignLights  Port=2  SampleTime=50/1000
  wires:
  GND1/1 -> VISUMatrixSign_HighwayOverhang_5/1
  GND2/1 -> VISUMatrixSignLights_HighwayOverhang_5/1

== system Demo_PreScanCarSim3D_ExtFMU_cs/HighwayOverhang_5/ENABLED ==
  note: Resources
      |
      | 3: InformationSign\MatrixSign_Empty.png: MatrixSign Empty
      | 4: InformationSign\MatrixSign_End.png: MatrixSign End
      | 5: InformationSign\MatrixSign_GreenArrow.png: MatrixSign GreenArrow
      | 6: InformationSign\MatrixSign_RedCross.png: MatrixSign RedCross
      | 7: InformationSign\MatrixSign_Speed_50.png: MatrixSign Speed 50
      | 8: InformationSign\MatrixSign_Speed_70.png: MatrixSign Speed 70
      | 9: InformationSign\MatrixSign_Speed_90.png: MatrixSign Speed 90
      | 10: InformationSign\MatrixSign_Speed_120.png: MatrixSign Speed 120
      | 11: InformationSign\MatrixSign_Speed_130.png: MatrixSign Speed 130
      | 12: InformationSign\information.png: information
      | 13: InformationSign\TASS-international-logo.bmp: TASS-international-logo
  Ground_{1..6} (6 alike) : Ground
  VISUMatrixSignLights_Mux : Subsystem  Tag=mux/VisuMatrixSignLights  mask(PreScan User Interface: VisuMatrixSignLights){}
      mask help:
      | The VisuMatrixSignLights block provides a way to switch the lights on the matrix sign board on or off
      |
      | For more information, please click Help.
      mask Help: eval('openHelp(732)')
  VISUMatrixSign_Mux : Subsystem  Tag=mux/MatrixSign_v2  mask(PreScan User Interface: VisuMatrixSign){}
      mask help:
      | The VisuMatrixSign block provides a way to adapt the texture of the plates connected to an overhang, based on Resource IDs of the texture files.
      |
      | For more information, please click Help.
      settings: DeleteFcn=PreScanBlockDeleteFcn;
      mask Help: eval('openHelp(733)')
  VISUMatrixSign_HighwayOverhang_5 : Outport  Tag=outport/VisuMatrixSign  SampleTime=50/1000
  VISUMatrixSignLights_HighwayOverhang_5 : Outport  Tag=outport/VisuMatrixSignLights  Port=2  SampleTime=50/1000
  wires:
  VISUMatrixSign_Mux/1(MatrixSigns) -> VISUMatrixSign_HighwayOverhang_5/1
  VISUMatrixSignLights_Mux/1(VISUMatrixSignLights_HighwayOverhang_5) -> VISUMatrixSignLights_HighwayOverhang_5/1
  Ground_1/1 -> VISUMatrixSignLights_Mux/1(MatrixSign_18)
  Ground_2/1 -> VISUMatrixSignLights_Mux/2(MatrixSign_19)
  Ground_3/1 -> VISUMatrixSignLights_Mux/3(MatrixSign_20)
  Ground_4/1 -> VISUMatrixSign_Mux/1(MatrixSign_18)
  Ground_5/1 -> VISUMatrixSign_Mux/2(MatrixSign_19)
  Ground_6/1 -> VISUMatrixSign_Mux/3(MatrixSign_20)

== system Demo_PreScanCarSim3D_ExtFMU_cs/SELF_Audi_A8_1/DISABLED ==
  GND1 : Subsystem
  SELF_Audi_A8_1 : Outport  Tag=outport/SelfPort  OutDataTypeStr=Bus: PRESCAN_SELFSENSORDATA  PortDimensions=1  SampleTime=50/1000
  wires:
  GND1/1(bus) -> SELF_Audi_A8_1/1

== system Demo_PreScanCarSim3D_ExtFMU_cs/SELF_Audi_A8_1/ENABLED ==
  Sensor : S-Function  FunctionName=sfun_SelfSensor  Parameters=UniqueID, TimeStep  SFunctionDeploymentMode=off  EnableBusSupport=off  mask(PreScan Source Block: SELF){UniqueID=3037, TimeStep=50/1000}
      mask prompts: UniqueID "Auto-Assigned: Unique ID"; TimeStep "Auto-Assigned: Upload Period [s]"
      mask help:
      | The SELF port shows (state) information of the actor itself. The outputs are position in the experiment's axis system and the GPS coordinates, and the object's absolute velocity and compass heading.
      |
      | For more information, please click Help.
      mask Help: eval('openHelp(462)')
      mask Display: image(imread('GPS.png'))
  SELF_Audi_A8_1 : Outport  Tag=outport/SelfPort  OutDataTypeStr=Bus: PRESCAN_SELFSENSORDATA  PortDimensions=1  SampleTime=50/1000
  wires:
  Sensor/1 -> SELF_Audi_A8_1/1

== system Demo_PreScanCarSim3D_ExtFMU_cs/SELF_Box_1/DISABLED ==
  GND1 : Subsystem
  SELF_Box_1 : Outport  Tag=outport/SelfPort  OutDataTypeStr=Bus: PRESCAN_SELFSENSORDATA  PortDimensions=1  SampleTime=50/1000
  wires:
  GND1/1(bus) -> SELF_Box_1/1

== system Demo_PreScanCarSim3D_ExtFMU_cs/SELF_Box_1/ENABLED ==
  Sensor : S-Function  FunctionName=sfun_SelfSensor  Parameters=UniqueID, TimeStep  SFunctionDeploymentMode=off  EnableBusSupport=off  mask(PreScan Source Block: SELF){UniqueID=2076, TimeStep=50/1000}
      mask prompts: UniqueID "Auto-Assigned: Unique ID"; TimeStep "Auto-Assigned: Upload Period [s]"
      mask help:
      | The SELF port shows (state) information of the actor itself. The outputs are position in the experiment's axis system and the GPS coordinates, and the object's absolute velocity and compass heading.
      |
      | For more information, please click Help.
      mask Help: eval('openHelp(462)')
      mask Display: image(imread('GPS.png'))
  SELF_Box_1 : Outport  Tag=outport/SelfPort  OutDataTypeStr=Bus: PRESCAN_SELFSENSORDATA  PortDimensions=1  SampleTime=50/1000
  wires:
  Sensor/1 -> SELF_Box_1/1

== system Demo_PreScanCarSim3D_ExtFMU_cs/SELF_Box_2/DISABLED ==
  GND1 : Subsystem
  SELF_Box_2 : Outport  Tag=outport/SelfPort  OutDataTypeStr=Bus: PRESCAN_SELFSENSORDATA  PortDimensions=1  SampleTime=50/1000
  wires:
  GND1/1(bus) -> SELF_Box_2/1

== system Demo_PreScanCarSim3D_ExtFMU_cs/SELF_Box_2/ENABLED ==
  Sensor : S-Function  FunctionName=sfun_SelfSensor  Parameters=UniqueID, TimeStep  SFunctionDeploymentMode=off  EnableBusSupport=off  mask(PreScan Source Block: SELF){UniqueID=2077, TimeStep=50/1000}
      mask prompts: UniqueID "Auto-Assigned: Unique ID"; TimeStep "Auto-Assigned: Upload Period [s]"
      mask help:
      | The SELF port shows (state) information of the actor itself. The outputs are position in the experiment's axis system and the GPS coordinates, and the object's absolute velocity and compass heading.
      |
      | For more information, please click Help.
      mask Help: eval('openHelp(462)')
      mask Display: image(imread('GPS.png'))
  SELF_Box_2 : Outport  Tag=outport/SelfPort  OutDataTypeStr=Bus: PRESCAN_SELFSENSORDATA  PortDimensions=1  SampleTime=50/1000
  wires:
  Sensor/1 -> SELF_Box_2/1

== system Demo_PreScanCarSim3D_ExtFMU_cs/SELF_Box_3/DISABLED ==
  GND1 : Subsystem
  SELF_Box_3 : Outport  Tag=outport/SelfPort  OutDataTypeStr=Bus: PRESCAN_SELFSENSORDATA  PortDimensions=1  SampleTime=50/1000
  wires:
  GND1/1(bus) -> SELF_Box_3/1

== system Demo_PreScanCarSim3D_ExtFMU_cs/SELF_Box_3/ENABLED ==
  Sensor : S-Function  FunctionName=sfun_SelfSensor  Parameters=UniqueID, TimeStep  SFunctionDeploymentMode=off  EnableBusSupport=off  mask(PreScan Source Block: SELF){UniqueID=2078, TimeStep=50/1000}
      mask prompts: UniqueID "Auto-Assigned: Unique ID"; TimeStep "Auto-Assigned: Upload Period [s]"
      mask help:
      | The SELF port shows (state) information of the actor itself. The outputs are position in the experiment's axis system and the GPS coordinates, and the object's absolute velocity and compass heading.
      |
      | For more information, please click Help.
      mask Help: eval('openHelp(462)')
      mask Display: image(imread('GPS.png'))
  SELF_Box_3 : Outport  Tag=outport/SelfPort  OutDataTypeStr=Bus: PRESCAN_SELFSENSORDATA  PortDimensions=1  SampleTime=50/1000
  wires:
  Sensor/1 -> SELF_Box_3/1

== system Demo_PreScanCarSim3D_ExtFMU_cs/SELF_Box_4/DISABLED ==
  GND1 : Subsystem
  SELF_Box_4 : Outport  Tag=outport/SelfPort  OutDataTypeStr=Bus: PRESCAN_SELFSENSORDATA  PortDimensions=1  SampleTime=50/1000
  wires:
  GND1/1(bus) -> SELF_Box_4/1

== system Demo_PreScanCarSim3D_ExtFMU_cs/SELF_Box_4/ENABLED ==
  Sensor : S-Function  FunctionName=sfun_SelfSensor  Parameters=UniqueID, TimeStep  SFunctionDeploymentMode=off  EnableBusSupport=off  mask(PreScan Source Block: SELF){UniqueID=2079, TimeStep=50/1000}
      mask prompts: UniqueID "Auto-Assigned: Unique ID"; TimeStep "Auto-Assigned: Upload Period [s]"
      mask help:
      | The SELF port shows (state) information of the actor itself. The outputs are position in the experiment's axis system and the GPS coordinates, and the object's absolute velocity and compass heading.
      |
      | For more information, please click Help.
      mask Help: eval('openHelp(462)')
      mask Display: image(imread('GPS.png'))
  SELF_Box_4 : Outport  Tag=outport/SelfPort  OutDataTypeStr=Bus: PRESCAN_SELFSENSORDATA  PortDimensions=1  SampleTime=50/1000
  wires:
  Sensor/1 -> SELF_Box_4/1
